simulink model "nonlinear_sim"  (R2025a)
settings: Solver=FixedStepAuto  StartTime=0.0  StopTime=30  FixedStep=dt_sim  RelTol=1e-3
values from neighbouring files (symbols this model uses):
  a = 1116.45    [gain_scheduled_controller_design.m]    (also in setup_data_for_DC_input_comparison_test.m)
  Actuator = dummy.SimPar_STRUCT.Actuator    [gain_scheduled_controller_design.m]    (also in setup_data_for_DC_input_comparison_test.m)
  Engine = dummy.SimPar_STRUCT.Engine    [gain_scheduled_controller_design.m]    (also in setup_data_for_DC_input_comparison_test.m)
  grav = 32.17405    [gain_scheduled_controller_design.m]    (also in setup_data_for_DC_input_comparison_test.m)
  init_eng_dyn = ueq(5:end)    [gain_scheduled_controller_design.m]    (also in setup_data_for_DC_input_comparison_test.m)
  init_surf_dyn = surf_alloc_mat * ueq(1:4)    [gain_scheduled_controller_design.m]    (also in setup_data_for_DC_input_comparison_test.m)
  init_x_eom = [init_euler; init_vbar; init_pqr]    [gain_scheduled_controller_design.m]    (also in setup_data_for_DC_input_comparison_test.m)
  J = lpc.I    [gain_scheduled_controller_design.m]    (also in setup_data_for_DC_input_comparison_test.m)
  m = lpc.mass    [gain_scheduled_controller_design.m]    (also in setup_data_for_DC_input_comparison_test.m)
  Model = lpc    [gain_scheduled_controller_design.m]    (also in setup_data_for_DC_input_comparison_test.m)
  rho = 0.00237717    [gain_scheduled_controller_design.m]    (also in setup_data_for_DC_input_comparison_test.m)
  surf_alloc_mat = [1, -1, 0, 0;                    1,  1, 0, 0;                    0,  0, 1, 0;                    0,  0, 1, 0;                    0,  0, 0, 1;]    [gain_scheduled_controller_design.m]    (also in setup_data_for_DC_input_comparison_test.m)
  u_trim = ueq    [setup_data_for_DC_input_comparison_test.m]
  Units = dummy.SimIn.Units    [gain_scheduled_controller_design.m]    (also in setup_data_for_DC_input_comparison_test.m)
undefined symbols (not defined in the file or in its folder): Kr_hover, Kx_hover, ref_cmd_STEP, ref_cmd_trim, x_trim
libraries: ServosLib x2
settings Model: Creator=alhallmark  LastModifiedBy=alhallmark

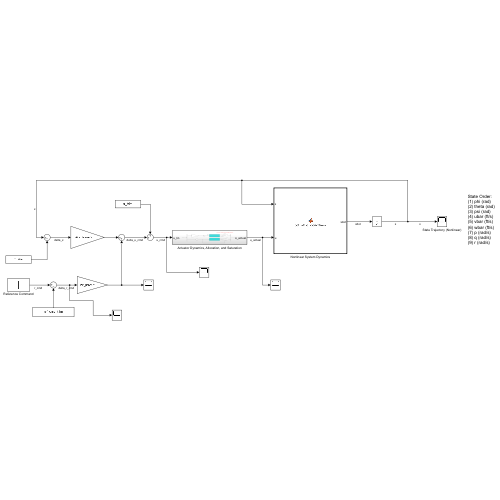
[thumbnail: Simulink's stored preview of the top-level diagram]
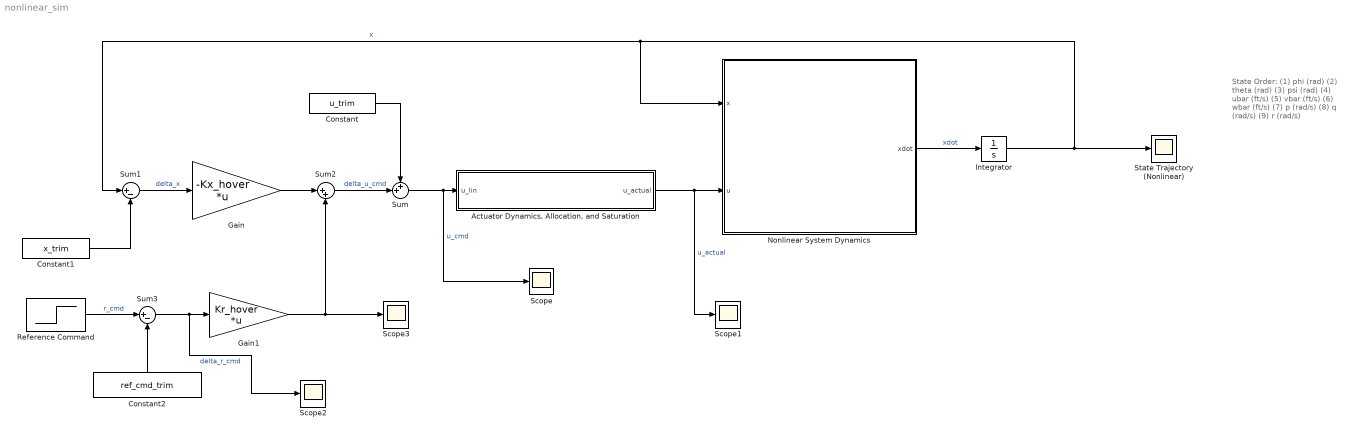
== system nonlinear_sim ==
  note: State Order:
      | (1) phi (rad)
      | (2) theta (rad)
      | (3) psi (rad)
      | (4) ubar (ft/s)
      | (5) vbar (ft/s)
      | (6) wbar (ft/s)
      | (7) p (rad/s)
      | (8) q (rad/s)
      | (9) r (rad/s)
  "Actuator Dynamics, Allocation, and Saturation" : Subsystem
  Constant : Constant  Value=u_trim
  Constant1 : Constant  Value=x_trim
  Constant2 : Constant  Value=ref_cmd_trim
  Gain : Gain  Gain=-Kx_hover  Multiplication=Matrix(K*u)
  Gain1 : Gain  Gain=Kr_hover  Multiplication=Matrix(K*u)
  Integrator : Integrator  InitialCondition=init_x_eom  ContinuousStateAttributes={'phi', 'theta', 'psi', 'ubar', 'vbar', 'wbar', 'p', 'q', 'r'}
  Nonlinear System Dynamics : MATLAB Function  TreatAsAtomicUnit=on
  Reference Command : Step  Before=[0; 0; 0]  After=ref_cmd_STEP  SampleTime=0
  Scope{,1..3} (4 alike) : Scope
      Scope settings: ActiveDisplayYMinimum=165.9697159388528  ActiveDisplayYMaximum=466.60829473365919
      Scope1 settings: ActiveDisplayYMinimum=-1  ActiveDisplayYMaximum=1  DataLoggingVariableName=ScopeData2
      Scope2 settings: ActiveDisplayYMinimum=-1.2499999999999998  ActiveDisplayYMaximum=11.25  DataLoggingVariableName=ScopeData3
      Scope3 settings: ActiveDisplayYMinimum=-1  ActiveDisplayYMaximum=1  DataLoggingVariableName=ScopeData4
  State Trajectory (Nonlinear) : Scope
      settings: ActiveDisplayYMinimum=-1.0123085975426203  ActiveDisplayYMaximum=2.8354423024556383
  Sum : Sum  Inputs=++|
  Sum1 : Sum  Inputs=|+-
  Sum2 : Sum  Inputs=|++
  Sum3 : Sum  Inputs=|+-
  wires:
  "Actuator Dynamics, Allocation, and Saturation"/1(u_actual) -> Nonlinear System Dynamics/2(u), Scope1/1  "u_actual"
  Sum/1 -> Scope/1, "Actuator Dynamics, Allocation, and Saturation"/1(u_lin)  "u_cmd"
  Nonlinear System Dynamics/1(xdot) -> Integrator/1  "xdot"
  Integrator/1 -> State Trajectory (Nonlinear)/1, Sum1/1, Nonlinear System Dynamics/1(x)  "x"
  Constant1/1 -> Sum1/2
  Sum1/1 -> Gain/1  "delta_x"
  Constant/1 -> Sum/1
  Sum2/1 -> Sum/2  "delta_u_cmd"
  Gain/1 -> Sum2/1
  Reference Command/1 -> Sum3/1  "r_cmd"
  Constant2/1 -> Sum3/2
  Sum3/1 -> Scope2/1, Gain1/1  "delta_r_cmd"
  Gain1/1 -> Sum2/2, Scope3/1

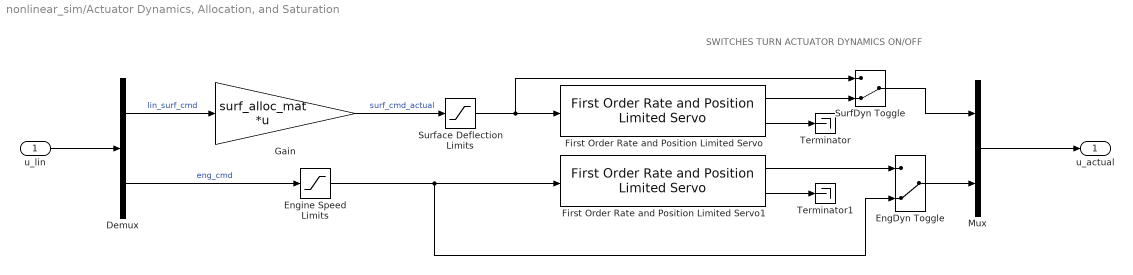
== system nonlinear_sim/Actuator Dynamics, Allocation, and Saturation ==
  note: SWITCHES TURN ACTUATOR DYNAMICS ON/OFF
  u_lin : Inport
  Demux : Demux  Outputs=[4, 9]
  EngDyn Toggle : ManualSwitch  CurrentSetting=0
  Engine Speed Limits : Saturate  UpperLimit=Engine.MaxPos  LowerLimit=Engine.MinPos
  First Order Rate and Position Limited Servo : ServosLib/First Order  Rate and Position Limited  Servo  freq=Actuator.BW  RL=Actuator.RL  POS_hi=Actuator.MaxPos  POS_lo=Actuator.MinPos  Bias=init_surf_dyn  StateName=ControlSurfaces
  First Order Rate and Position Limited Servo1 : ServosLib/First Order  Rate and Position Limited  Servo  freq=Engine.BW  RL=Engine.RL  POS_hi=Engine.MaxPos  POS_lo=Engine.MinPos  Bias=init_eng_dyn  StateName=EngineSpeed
  Gain : Gain  Gain=surf_alloc_mat  Multiplication=Matrix(K*u)
  Mux : Mux  Inputs=2
  SurfDyn Toggle : ManualSwitch  CurrentSetting=0
  Surface Deflection Limits : Saturate  UpperLimit=Actuator.MaxPos  LowerLimit=Actuator.MinPos
  Terminator : Terminator
  Terminator1 : Terminator
  u_actual : Outport
  wires:
  u_lin/1 -> Demux/1
  Demux/1 -> Gain/1  "lin_surf_cmd"
  Demux/2 -> Engine Speed Limits/1  "eng_cmd"
  Gain/1 -> Surface Deflection Limits/1  "surf_cmd_actual"
  Surface Deflection Limits/1 -> SurfDyn Toggle/1, First Order Rate and Position Limited Servo/1
  First Order Rate and Position Limited Servo/2 -> Terminator/1
  Mux/1 -> u_actual/1
  First Order Rate and Position Limited Servo/1 -> SurfDyn Toggle/2
  SurfDyn Toggle/1 -> Mux/1
  Engine Speed Limits/1 -> EngDyn Toggle/2, First Order Rate and Position Limited Servo1/1
  First Order Rate and Position Limited Servo1/2 -> Terminator1/1
  First Order Rate and Position Limited Servo1/1 -> EngDyn Toggle/1
  EngDyn Toggle/1 -> Mux/2

== matlab function nonlinear_sim/Nonlinear System Dynamics ==
  data: x input; u input; xdot output; J parameter; m parameter; grav parameter; rho parameter; a parameter; Units parameter; Model parameter
function xdot = get_state_derivatives(x, u, J, m, grav, rho, a, Units, Model)
% FUNCTION DOCUMENTATION:
%
% INPUTS:
%
% x : 9x1 state vector with order:
%
% [1] phi   : roll angle (radians)
% [2] theta : pitch angle (radians)
% [3] psi   : yaw angle (radians)
% [4] u_bar : x-velocity in heading frame (ft/s)
% [5] v_bar : y-velocity in heading frame (ft/s)
% [6] w_bar : z-velocity in heading frame (ft/s)
% [7] p : x-component of angular velocity vector (rad/s)
% [8] q : y-component of angular velocity vector (rad/s)
% [9] r : z-component of angular velocity vector (rad/s)
%
% u : 14x1 input vector with order:
% 
% [1] del_aL : left  aileron deflection (radians)
% [2] del_aR : right aileron deflection (radians)
% [3] del_eL : left  elevator deflection (radians)
% [4] del_eR : right elevator deflection (radians)
% [5] del_r  : rudder deflection (radians)
% [6]  om1   : prop 1 speed - rotor 1 (rad/s)
% [7]  om2   : prop 2 speed - rotor 2 (rad/s)
% [8]  om3   : prop 3 speed - rotor 3 (rad/s)
% [9]  om4   : prop 4 speed - rotor 4 (rad/s)
% [10] om5   : prop 5 speed - rotor 5 (rad/s)
% [11] om6   : prop 6 speed - rotor 6 (rad/s)
% [12] om7   : prop 7 speed - rotor 7 (rad/s)
% [13] om8   : prop 8 speed - rotor 8 (rad/s)
% [14] om9   : prop 9 speed - pusher  (rad/s)
% 
% J (parameter data) : vehicle inertia matrix in body frame (slug*ft^2 ?)
% m (parameter data) : vehicle mass (slug?)
% grav (parameter data) : acceleration due to gravity (ft/s^2)
% rho (parameter data) : air density @ SL (slug/ft^3)
% a (parameter data) : speed of sound @ SL (ft/s)
% Units (parameter data) : struct containing unit conversions (GUAM)
% Model (parameter data) : struct containing aircraft model info (GUAM)
%
% OUTPUTS:
% 
% xdot: time derivatives of the state vector (order same as x above -- the
% units are the same as x above but multiplied by 1/sec because of the
% differentiation w.r.t. time)
%
% NOTES:
% This function implements the dynamics (EOM) shown in section III.C of
% the 2021 SciTech paper "Examination of uniﬁed control approaches
% incorporating generalized control allocation" by Acheson et. al. : 

% Calculate/assign intermediate variables:
phi = x(1); % roll angle (rad)
theta = x(2); % pitch angle (rad)
omega_b = x(end-2:end); % 3x1 angular velocity in body frame (rad/s)
vbar = x(4:6); % velocity in heading frame (ft/s)

grav_vec = grav * [0; 0; 1]; % gravity vector in the heading frame 

% Calculate matrix relating the angular velocities to the euler rates:
S = [1, sin(phi)*tan(theta), cos(phi)*tan(theta); ...
     0, cos(phi), -sin(phi); ...
     0, sin(phi)/cos(theta), cos(phi)/cos(theta)];

euler_rates = S*omega_b; % get time derivatives of euler angles (rad/s)

psi_dot = euler_rates(3); % extract time derivative of yaw angle (rad/s)

% Get rotation matrix from the body frame to the heading frame:
R_bar = (rotx(rad2deg(phi)).' * roty(rad2deg(theta)).').';
% NOTE: the above matrix is defined such that v_heading = R_bar * v_body

% Get body frame velocity (needed for calling aeropropulsive model)
v_body = R_bar.' * vbar;

% Set up inputs for calling the aeropropulsive model:
x_aeroprop = [v_body; omega_b];
n_aeroprop = u(6:14);
d_aeroprop = u(1:5);

% Call the aeropropulsive model to get the 'external' aerodynamic and
% propulsive forces/moments in the body frame as a function of the current
% state and the current inputs:
[Fb, Mb, Validity] = run_LpC_aero(x_aeroprop, n_aeroprop, d_aeroprop, ...
    rho, a, Units, Model);

% Rotate the aeropropulsive force vector from the body-fixed frame to the
% heading frame:
F_heading_frame = R_bar * Fb;

% Calculate the time derivative of the velocity in the heading frame:
vbar_dot = -cross(psi_dot*[0; 0; 1], vbar) + grav_vec + ...
    (1/m) * F_heading_frame;

% Calculate the time derivative of the angular velocity (of the body-fixed 
% frame w.r.t. the inertial frame, expressed in the body-fixed frame):
omega_b_dot = J \ (-cross(omega_b, J*omega_b) + Mb);

xdot = [euler_rates; vbar_dot; omega_b_dot];

end
